simulink model "project1_lib_updated_2016b"  (R2016b)
settings: Solver=ode2  StartTime=0.0  StopTime=4000  FixedStep=1  RelTol=1e-3  EnableMultiTasking=on
undefined symbols (not defined in the file or in its folder): eng_map, param
settings Model: Creator=wasynczu  LastModifiedBy=wasynczu
settings DataIOCC: LimitDataPoints=on  SaveFormat=Array
settings OptimizationCC: LifeSpan=inf
settings DebuggingCC: SolverPrmCheckMsg=warning  AllowSymbolicDim=off  SFUnexpectedBacktrackingDiag=warning  SFNoUnconditionalDefaultTransitionDiag=warning  SFExecutionAtInitializationDiag=none
settings HardwareCC: ProdBitPerPointer=32  ProdBitPerSizeT=32  ProdBitPerPtrDiffT=32  ProdLargestAtomicFloat=None  ProdIntDivRoundTo=Undefined  ProdEndianess=Unspecified  ProdWordSize=32  ProdHWDeviceType=32-bit Generic
settings ModelReferenceCC: PropagateSignalLabelsOutOfModel=off
settings GRTTargetCC: TargetLangStandard=C89/C90 (ANSI)
settings ConfigComp: CovMetricSettings=dw  CovHtmlReporting=on  CovSaveCumulativeToWorkspaceVar=on  CovSaveSingleToWorkspaceVar=on  CovExternalEMLEnable=off  CovSFcnEnable=off

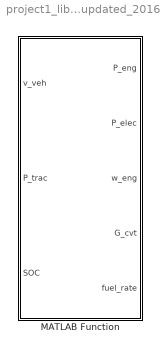
== system project1_lib_updated_2016b ==
  MATLAB Function : MATLAB Function  TreatAsAtomicUnit=on

== matlab function project1_lib_updated_2016b/MATLAB Function ==
  data: v_veh input; P_eng output; P_trac input; SOC input; P_elec output; w_eng output; G_cvt output; fuel_rate output; param parameter; eng_map parameter
function [P_eng, P_elec, w_eng, G_cvt, fuel_rate] = fcn(v_veh, P_trac, SOC, param, eng_map)
%#codegen
%inputs:
    % v_veh, m/s
    % P_trac, W
    % SOC
    % param, structure of parameters
    % eng_map

% outputs:
    %   P_gen, P_elec in W
    %   w_eng, rpm
    %   G_cvt (cvt ratio)
    %   Fuel rate, g/hr

v_veh_min = param.v_veh_min;    % minimum vehicle speed for engine to stay engaged, in m/s
P_eng_min = param.P_eng_min;    % minimum engine power in W
P_eng_max = param.P_eng_max ;   % maximum engine power
G_cvt_min = param.G_cvt_min;    % minimum cvt  ratio
G_diff = param.G_diff;          % differential gear ratio
r_wheel = param.r_wheel;        % wheel radius in m

if (v_veh < v_veh_min)  % disengage clutch, idle, engine, electric launch
   P_elec = P_trac;
   P_eng = 0;
   fuel_rate = 0; % g/hr;
   w_eng = 0; % rpm
   G_cvt = G_cvt_min;
   return  
end

% if here, v_veh > v_veh_min
if(P_trac < P_eng_min)   % clutch engaged but no fuel
   P_elec = P_trac;
   fuel_rate = 0;
   P_eng = 0;
   w_eng =  1000; % rpm
   w_eng_SI = w_eng * 2 * pi / 60; % rad/s
   % set G_cvt so engine speed is 1000 rpm
   G_cvt = v_veh/G_diff/w_eng_SI/r_wheel;
   return     
end

if(P_trac > P_eng_max) % high-speed boost
   P_elec = P_trac - P_eng_max;
   P_eng = P_eng_max;
   bsfc = interp1(eng_map(:,2), eng_map(:,3), P_eng/1000);
   fuel_rate = bsfc*P_eng/1000; % g/hr
   w_eng = interp1(eng_map(:,2), eng_map(:,1), P_eng/1000);
   w_eng_SI = w_eng * 2 * pi / 60; % convert to rad/s
   G_cvt =  v_veh/r_wheel/G_diff/w_eng_SI; % required CVT ratio
   return   
end

% if here, v_veh > v_veh_min and P_eng_min < P_trac < P_eng_max
% try to get SOC back to 0.5

P_elec = 4000*sign(SOC - 0.5); 
P_eng = P_trac - P_elec;

if(P_eng < P_eng_min) 
   % clutch engaged, but no fuel
   P_eng = 0;
   P_elec = P_trac;
   fuel_rate = 0;
   w_eng = 1000;
   w_eng_SI = w_eng * 2 * pi / 60; % om rad/s
   % set G_cvt so engine speed is 1000 rpm
   G_cvt = v_veh/G_diff/w_eng_SI/r_wheel;
   return
end

if(P_eng > P_eng_max)
    P_eng = P_eng_max;
    P_elec = P_trac - P_eng_max;
end

bsfc = interp1(eng_map(:,2), eng_map(:,3), P_eng/1000);
fuel_rate = bsfc*P_eng/1000; % g/hr

w_eng = interp1(eng_map(:,2), eng_map(:,1), P_eng/1000);
w_eng_SI = w_eng* pi / 30;  % convert to rad/s
G_cvt =  v_veh/r_wheel/G_diff/w_eng_SI;

if (G_cvt < G_cvt_min) % set G_cvt = G_cvt_min, recalculate w_eng, P_eng, and P_elec
   G_cvt = G_cvt_min;
   w_eng_SI = v_veh/G_diff/r_wheel/G_cvt;
   w_eng = w_eng_SI*30/pi;  % in rpm
   P_eng = 1000*interp1(eng_map(:,1), eng_map(:,2), w_eng) % in W
   P_elec = P_trac - P_eng;
   bsfc = interp1(eng_map(:,1), eng_map(:,3), w_eng);
   fuel_rate = bsfc*P_eng/1000; % g/hr
 end
